simulink library "Simple_lib"  (R2018b)
settings: Solver=ode45  StartTime=0.0  StopTime=10.0  RelTol=1e-3  EnableMultiTasking=on
undefined symbols (not defined in the file or in its folder): Acceptance, beta, C, C_J, C_P, c_wall, dGain, DiscIntNeverNeededParam, Duplex, Electrical_lib, grab, h_fe, i, i3, K_T, Kman, KmanCE, mu_s, n_rev, R_arm, Simplex, systemTs, tau_0, TinIC, Ts, w_0, wallMass, Watch_lib
libraries: $bdroot x407, PlantUtilityBlockset_lib x30, peGeneralControl x22, simulink x11
(part 14 of 14)

== system Simple_lib/Hydraulic/X Heat Exchanger/Pipe1/Pull ==
  InPot : Inport  Tag=NOFLUX
  FlowDisplay : Display
  FlowGain : Gain
  FlowSum : Sum  Inputs=2  SaturateOnIntegerOverflow=on  InputSameDT=on  OutDataTypeStr=Inherit: Same as first input
  Flow_PullO1BoxIIValveHydroNonStandard : Scope
      settings: Tag=Flow
  PotDisplay : Display
  Pot_PullO1BoxIIValveHydroNonStandard : Scope
      settings: Tag=Pot
  Rate Transition : RateTransition  OutPortSampleTimeMultiple=nT  OutPortSampleTime=Ts
  OutPot : Outport
  OutFlow : Outport  Tag=NOFLUX  Port=2
  wires:
  [PushInertiaChamber1CylinderHydroNonStandard] -> FlowSum/2
  [PushO3BoxXValveHydroNonStandard] -> FlowSum/1
  FlowSum/1 -> FlowGain/1
  FlowGain/1 -> FlowDisplay/1, Flow_PullO1BoxIIValveHydroNonStandard/1, OutFlow/1
  InPot/1 -> Pot_PullO1BoxIIValveHydroNonStandard/1, PotDisplay/1, Rate Transition/1
  Rate Transition/1 -> OutPot/1

== system Simple_lib/Hydraulic/X Heat Exchanger/Pipe1/Push ==
  InPot : Inport
  InFlow : Inport  Tag=NOFLUX  Port=2
  FlowDisplay : Display
  Flow_PushO1BoxIIValveHydroNonStandard : Scope
      settings: Tag=Flow
  PotDisplay : Display
  Pot_PushO1BoxIIValveHydroNonStandard : Scope
      settings: Tag=Pot
  Rate Transition : RateTransition  OutPortSampleTimeMultiple=Ts  OutPortSampleTime=Ts
  OutPot : Outport  Tag=NOFLUX
  tag scope: PushO1BoxIIValveHydroNonStandard=global
  wires:
  InPot/1 -> Rate Transition/1
  InFlow/1 -> Flow_PushO1BoxIIValveHydroNonStandard/1, FlowDisplay/1, [PushO1BoxIIValveHydroNonStandard]
  Rate Transition/1 -> OutPot/1, Pot_PushO1BoxIIValveHydroNonStandard/1, PotDisplay/1

== system Simple_lib/Hydraulic/X Heat Exchanger/Pipe2/Pull ==
  InPot : Inport  Tag=NOFLUX
  FlowDisplay : Display
  FlowGain : Gain
  FlowSum : Sum  Inputs=2  SaturateOnIntegerOverflow=on  InputSameDT=on  OutDataTypeStr=Inherit: Same as first input
  Flow_PullO1BoxIIValveHydroNonStandard : Scope
      settings: Tag=Flow
  PotDisplay : Display
  Pot_PullO1BoxIIValveHydroNonStandard : Scope
      settings: Tag=Pot
  Rate Transition : RateTransition  OutPortSampleTimeMultiple=nT  OutPortSampleTime=Ts
  OutPot : Outport
  OutFlow : Outport  Tag=NOFLUX  Port=2
  wires:
  [PushInertiaChamber1CylinderHydroNonStandard] -> FlowSum/2
  [PushO3BoxXValveHydroNonStandard] -> FlowSum/1
  FlowSum/1 -> FlowGain/1
  FlowGain/1 -> FlowDisplay/1, Flow_PullO1BoxIIValveHydroNonStandard/1, OutFlow/1
  InPot/1 -> Pot_PullO1BoxIIValveHydroNonStandard/1, PotDisplay/1, Rate Transition/1
  Rate Transition/1 -> OutPot/1

== system Simple_lib/Hydraulic/X Heat Exchanger/Pipe2/Push ==
  InPot : Inport
  InFlow : Inport  Tag=NOFLUX  Port=2
  FlowDisplay : Display
  Flow_PushO1BoxIIValveHydroNonStandard : Scope
      settings: Tag=Flow
  PotDisplay : Display
  Pot_PushO1BoxIIValveHydroNonStandard : Scope
      settings: Tag=Pot
  Rate Transition : RateTransition  OutPortSampleTimeMultiple=Ts  OutPortSampleTime=Ts
  OutPot : Outport  Tag=NOFLUX
  tag scope: PushO1BoxIIValveHydroNonStandard=global
  wires:
  InPot/1 -> Rate Transition/1
  InFlow/1 -> Flow_PushO1BoxIIValveHydroNonStandard/1, FlowDisplay/1, [PushO1BoxIIValveHydroNonStandard]
  Rate Transition/1 -> OutPot/1, Pot_PushO1BoxIIValveHydroNonStandard/1, PotDisplay/1

== system Simple_lib/Junkyard/CinWall/C/Duplex ==
  InPot : Inport  Tag=NOFLUX
  FlowDisplay : Display
  FlowGain : Gain
  FlowSum : Sum  Inputs=2  SaturateOnIntegerOverflow=on  InputSameDT=on  OutDataTypeStr=Inherit: Same as first input
  Flow_DuplexCCinWallHouseWithIcons : Scope
      settings: Tag=Flow
  PotDisplay : Display
  Pot_DuplexCCinWallHouseWithIcons : Scope
      settings: Tag=Pot
  Rate Transition : RateTransition  OutPortSampleTimeMultiple=nT  OutPortSampleTime=Ts
  OutPot : Outport
  OutFlow : Outport  Tag=NOFLUX  Port=2
  wires:
  [SimplexR17HouseWithIcons] -> FlowSum/2
  [Simplex1h_W_AtmHouseWithIcons] -> FlowSum/1
  FlowSum/1 -> FlowGain/1
  FlowGain/1 -> FlowDisplay/1, Flow_DuplexCCinWallHouseWithIcons/1, OutFlow/1
  InPot/1 -> Pot_DuplexCCinWallHouseWithIcons/1, PotDisplay/1, Rate Transition/1
  Rate Transition/1 -> OutPot/1

== system Simple_lib/Junkyard/CinWall/C/Simplex ==
  InPot : Inport
  InFlow : Inport  Tag=NOFLUX  Port=2
  FlowDisplay : Display
  Flow_SimplexCCinWallHouseWithIcons : Scope
      settings: Tag=Flow
  PotDisplay : Display
  Pot_SimplexCCinWallHouseWithIcons : Scope
      settings: Tag=Pot
  Rate Transition : RateTransition  OutPortSampleTimeMultiple=Ts  OutPortSampleTime=Ts
  OutPot : Outport  Tag=NOFLUX
  tag scope: SimplexCCinWallHouseWithIcons=global
  wires:
  InPot/1 -> Rate Transition/1
  InFlow/1 -> Flow_SimplexCCinWallHouseWithIcons/1, FlowDisplay/1, [SimplexCCinWallHouseWithIcons]
  Rate Transition/1 -> OutPot/1, Pot_SimplexCCinWallHouseWithIcons/1, PotDisplay/1

== system Simple_lib/Junkyard/CinWall/Gnd/Duplex ==
  InPot : Inport  Tag=NOFLUX
  FlowDisplay : Display
  FlowGain : Gain
  Flow_DuplexGndCinWallHouseWithIcons : Scope
      settings: Tag=Flow
  PotDisplay : Display
  Pot_DuplexGndCinWallHouseWithIcons : Scope
      settings: Tag=Pot
  Rate Transition : RateTransition  OutPortSampleTimeMultiple=nT  OutPortSampleTime=Ts
  OutPot : Outport
  OutFlow : Outport  Tag=NOFLUX  Port=2
  wires:
  [SimplexCCinWallHouseWithIcons] -> FlowGain/1
  FlowGain/1 -> FlowDisplay/1, Flow_DuplexGndCinWallHouseWithIcons/1, OutFlow/1
  InPot/1 -> Pot_DuplexGndCinWallHouseWithIcons/1, PotDisplay/1, Rate Transition/1
  Rate Transition/1 -> OutPot/1

== system Simple_lib/Thermal/CinWall/C/Duplex ==
  InPot : Inport  Tag=NOFLUX
  FlowDisplay : Display
  FlowGain : Gain
  FlowSum : Sum  Inputs=2  SaturateOnIntegerOverflow=on  InputSameDT=on  OutDataTypeStr=Inherit: Same as first input
  Flow_DuplexCCinWallHouseWithIcons : Scope
      settings: Tag=Flow
  PotDisplay : Display
  Pot_DuplexCCinWallHouseWithIcons : Scope
      settings: Tag=Pot
  Rate Transition : RateTransition  OutPortSampleTimeMultiple=nT  OutPortSampleTime=Ts
  OutPot : Outport
  OutFlow : Outport  Tag=NOFLUX  Port=2
  wires:
  [SimplexR17HouseWithIcons] -> FlowSum/2
  [Simplex1h_W_AtmHouseWithIcons] -> FlowSum/1
  FlowSum/1 -> FlowGain/1
  FlowGain/1 -> FlowDisplay/1, Flow_DuplexCCinWallHouseWithIcons/1, OutFlow/1
  InPot/1 -> Pot_DuplexCCinWallHouseWithIcons/1, PotDisplay/1, Rate Transition/1
  Rate Transition/1 -> OutPot/1

== system Simple_lib/Thermal/CinWall/C/Simplex ==
  InPot : Inport
  InFlow : Inport  Tag=NOFLUX  Port=2
  FlowDisplay : Display
  Flow_SimplexCCinWallHouseWithIcons : Scope
      settings: Tag=Flow
  PotDisplay : Display
  Pot_SimplexCCinWallHouseWithIcons : Scope
      settings: Tag=Pot
  Rate Transition : RateTransition  OutPortSampleTimeMultiple=Ts  OutPortSampleTime=Ts
  OutPot : Outport  Tag=NOFLUX
  tag scope: SimplexCCinWallHouseWithIcons=global
  wires:
  InPot/1 -> Rate Transition/1
  InFlow/1 -> Flow_SimplexCCinWallHouseWithIcons/1, FlowDisplay/1, [SimplexCCinWallHouseWithIcons]
  Rate Transition/1 -> OutPot/1, Pot_SimplexCCinWallHouseWithIcons/1, PotDisplay/1

== system Simple_lib/Thermal/CinWall/Gnd/Duplex ==
  InPot : Inport  Tag=NOFLUX
  FlowDisplay : Display
  FlowGain : Gain
  Flow_DuplexGndCinWallHouseWithIcons : Scope
      settings: Tag=Flow
  PotDisplay : Display
  Pot_DuplexGndCinWallHouseWithIcons : Scope
      settings: Tag=Pot
  Rate Transition : RateTransition  OutPortSampleTimeMultiple=nT  OutPortSampleTime=Ts
  OutPot : Outport
  OutFlow : Outport  Tag=NOFLUX  Port=2
  wires:
  [SimplexCCinWallHouseWithIcons] -> FlowGain/1
  FlowGain/1 -> FlowDisplay/1, Flow_DuplexGndCinWallHouseWithIcons/1, OutFlow/1
  InPot/1 -> Pot_DuplexGndCinWallHouseWithIcons/1, PotDisplay/1, Rate Transition/1
  Rate Transition/1 -> OutPot/1

== system Simple_lib/Driveline/Changan Transmission/EMachine/J_eMotor/Pull ==
  InPot : Inport  Tag=NOFLUX
  FlowGain : Gain
  FlowSum : Sum  Inputs=4  SaturateOnIntegerOverflow=on  InputSameDT=on  OutDataTypeStr=Inherit: Same as first input
  OutPot : Outport
  OutFlow : Outport  Tag=NOFLUX  Port=2
  wires:
  InPot/1 -> OutPot/1  "p_DuplexInverter_test0"
  FlowGain/1 -> OutFlow/1  "f_DuplexInverter_test0"
  FlowSum/1 -> FlowGain/1
  [SimplexTransducerEMachineTransmissionHYBPTPlantHybpt_test] -> FlowSum/1
  [Push_outK0TransmissionHYBPTPlantHybpt_test] -> FlowSum/2
  [Push_inK1TransmissionHYBPTPlantHybpt_test] -> FlowSum/3
  [Push_inK2TransmissionHYBPTPlantHybpt_test] -> FlowSum/4

== system Simple_lib/Driveline/Changan Transmission/EMachine/Transducer/Duplex ==
  InPot : Inport  Tag=NOFLUX
  FlowGain : Gain
  OutPot : Outport
  OutFlow : Outport  Tag=NOFLUX  Port=2
  wires:
  FlowGain/1 -> OutFlow/1  "out_DuplexTransducerEFADBEVPlantBEV"
  InPot/1 -> OutPot/1  "DuplexTransducerEFADBEVPlantBEV"
  [SimplexRDCDCHYBPTPlantHybpt_test] -> FlowGain/1

== system Simple_lib/Driveline/Changan Transmission/EMachine/Transducer/Simplex ==
  InPot : Inport
  InFlow : Inport  Tag=NOFLUX  Port=2
  OutPot : Outport  Tag=NOFLUX
  tag scope: SimplexTransducerEMachineTransmissionHYBPTPlantHybpt_test=global
  wires:
  InPot/1 -> OutPot/1  "SimplexTransducerEFADBEVPlantBEV"
  InFlow/1 -> [SimplexTransducerEMachineTransmissionHYBPTPlantHybpt_test]  "out_SimplexTransducerEFADBEVPlantBEV"
